simulink model "poleplacement_2"  (Simulink 7.8)
settings: Solver=ode1  StartTime=0.0  StopTime=inf  FixedStep=0.002  RelTol=1e-3
values from neighbouring files (symbols this model uses):
  k_1 = K(1)    [lqr_lab.m]
  k_2 = K(2)    [lqr_lab.m]
  k_3 = K(3)    [lqr_lab.m]
  k_4 = K(4)    [lqr_lab.m]
  Kth = 0.00153    [params.m]
  Kx = 2.28E-5    (= 2.28e-05)    [params.m]
undefined symbols (not defined in the file or in its folder): HIL
libraries: quarc_library x3, dsparch4 x2, simulink_extras x1
settings Model: Creator=dlavoi14  LastModifiedBy=dlavoi14  SimulationMode=external  ExtModeTrigDuration=5000
settings SolverCC: PositivePriorityOrder=on
settings RTWCC: SystemTargetFile=quarc_win64.tlc  TemplateMakefile=quarc_default_tmf  Description=QUARC Win64 Target  ProcessScript=quarc_win64_make_rtw_hook
settings STFCustomTargetCC: TargetPreCompLibLocation=C:\PROGRA~3\QUARC\lib\2011b\win64\release  SystemTargetFile=quarc_win64.tlc
settings GRTTargetCC: TargetPreCompLibLocation=C:\PROGRA~3\QUARC\lib\2011b\win64\release  ParMdlRefBuildCompliant=off  CompOptLevelCompliant=off  ConcurrentExecutionCompliant=off  MatFileLogging=off  ExtMode=on  ExtModeMexFile=quarc_comm

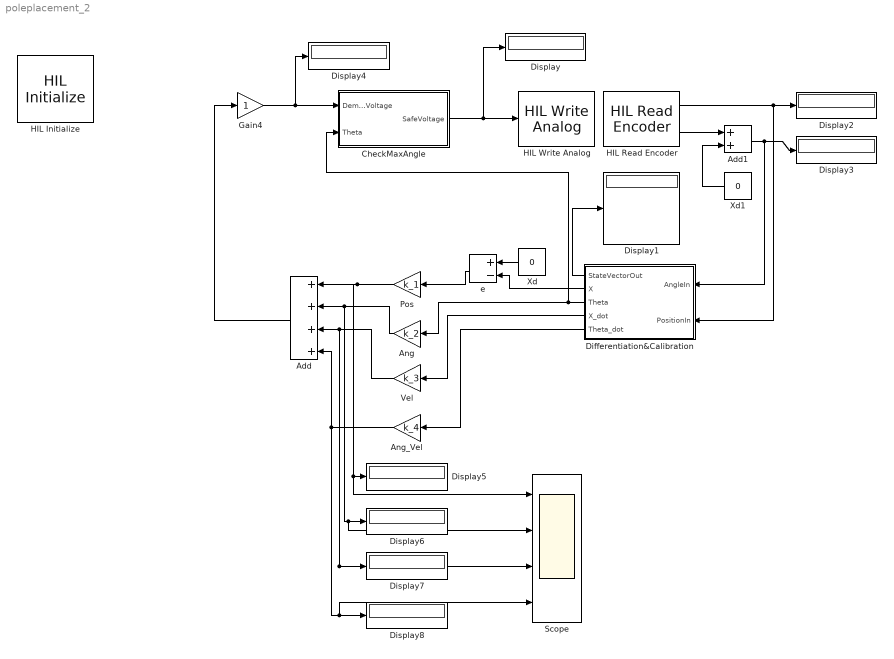
== system poleplacement_2 ==
  Add : Sum  Inputs=++++
  Add1 : Sum
  Ang : Gain  Gain=k_2
  Ang_Vel : Gain  Gain=k_4
  CheckMaxAngle : Subsystem
  Differentiation&Calibration : Subsystem
  Display{,1..8} (9 alike) : Display
  Gain4 : Gain
  HIL Initialize : quarc_library/Data Acquisition/Generic/Configuration/HIL Initialize  Priority=-99  object_name=HIL-1  board_type=q4  board_number=0  exclusive=off  active=off  hardware_clocks=[0:1]  clock_modes=[0 0]  initial_clock_frequencies=[]  set_clock_params_at_start=on  set_clock_params_at_switch_in=off  set_clock_frequencies_at_start=off  set_clock_frequencies_at_switch_in=off  analog_input_channels=[0:3]  analog_input_maximums=10  analog_input_minimums=-10  set_analog_input_params_at_start=off  set_analog_input_params_at_switch_in=off  analog_output_channels=[0:3]  analog_output_maximums=[10]  analog_output_minimums=[-10]  initial_analog_outputs=[0]  final_analog_outputs=[0]  watchdog_analog_outputs=0  set_analog_output_params_at_start=on  set_analog_output_params_at_switch_in=off  set_analog_outputs_at_start=on  set_analog_outputs_at_switch_in=off  set_analog_outputs_at_terminate=on  set_analog_outputs_at_switch_out=off  set_analog_outputs_on_watchdog=off  digital_input_channels=[]  digital_output_channels=[]  digital_output_configuration=[]  initial_digital_outputs=[1]  final_digital_outputs=[1]  watchdog_digital_outputs=[2]  set_digital_output_params_at_start=off  set_digital_output_params_at_switch_in=off  set_digital_outputs_at_start=on  set_digital_outputs_at_switch_in=off  set_digital_outputs_at_terminate=on  set_digital_outputs_at_switch_out=off  set_digital_outputs_on_watchdog=off  encoder_channels=[0:3]  quadrature=[4]  encoder_filter_frequency=(1/60e-9)/1  initial_encoder_counts=[0]  set_encoder_params_at_start=on  set_encoder_params_at_switch_in=off  set_encoder_counts_at_start=on  set_encoder_counts_at_switch_in=off  pwm_channels=[]  pwm_modes=[0]  pwm_frequency=(1/60e-9)/1024  pwm_configuration=[]  pwm_alignment=[]  pwm_polarity=[]  pwm_leading_deadband=[]  pwm_trailing_deadband=[]  initial_pwm_outputs=[0]  final_pwm_outputs=[0]  watchdog_pwm_outputs=[]  set_pwm_params_at_start=on  set_pwm_params_at_switch_in=off  set_pwm_outputs_at_start=on  set_pwm_outputs_at_switch_in=off  set_pwm_outputs_at_terminate=on  set_pwm_outputs_at_switch_out=off  set_pwm_outputs_on_watchdog=off  other_output_channels=[]  initial_other_outputs=[]  final_other_outputs=[]  watchdog_other_outputs=[]  set_other_outputs_at_start=off  set_other_outputs_at_switch_in=off  set_other_outputs_at_terminate=off  set_other_outputs_at_switch_out=off  set_other_outputs_on_watchdog=off
  HIL Read Encoder : quarc_library/Data Acquisition/Generic/Immediate I//O/HIL Read Encoder  object_name=HIL-1  channels=[0:1]  sample_time=qc_get_step_size  active=on  vector_output=off  data_type_mode=Inherit via back propagation  data_type=double
  HIL Write Analog : quarc_library/Data Acquisition/Generic/Immediate I//O/HIL Write Analog  object_name=HIL-1  channels=0  sample_time=-1  active=off  vector_input=off
  Pos : Gain  Gain=k_1
  Scope : Scope  NumInputPorts=4
      settings: YMin=-5~-80~-22.5~-80  YMax=6~90~22.5~60
  Vel : Gain  Gain=k_3
  Xd : Constant  Value=0
  Xd1 : Constant  Value=0
  e : Sum  Inputs=+-
  wires:
  CheckMaxAngle/1(SafeVoltage) -> Display/1, HIL Write Analog/1
  HIL Read Encoder/1 -> Differentiation&Calibration/2(PositionIn), Display2/1
  Differentiation&Calibration/3(Theta) -> Ang/1, CheckMaxAngle/2(Theta)
  Differentiation&Calibration/4(X_dot) -> Vel/1
  Differentiation&Calibration/5(Theta_dot) -> Ang_Vel/1
  Pos/1 -> Add/1, Display5/1, Scope/1
  Ang/1 -> Add/2, Display6/1, Scope/2
  Vel/1 -> Add/3, Display7/1, Scope/3
  Ang_Vel/1 -> Add/4, Display8/1, Scope/4
  Add/1 -> Gain4/1
  Gain4/1 -> Display4/1, CheckMaxAngle/1(DemandedControlVoltage)
  Differentiation&Calibration/2(X) -> e/2
  e/1 -> Pos/1
  Xd/1 -> e/1
  HIL Read Encoder/2 -> Add1/1
  Xd1/1 -> Add1/2
  Add1/1 -> Display3/1, Differentiation&Calibration/1(AngleIn)
  Differentiation&Calibration/1(StateVectorOut) -> Display1/1

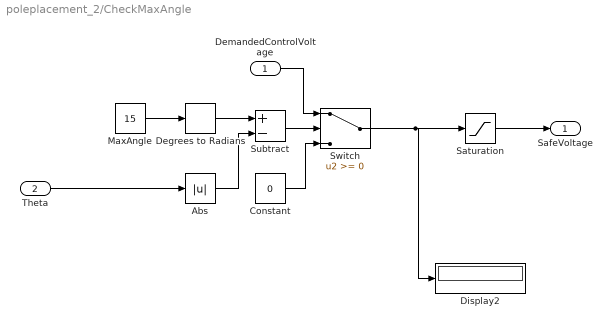
== system poleplacement_2/CheckMaxAngle ==
  DemandedControlVoltage : Inport
  Theta : Inport  Port=2
  Abs : Abs
  Constant : Constant  Value=0
  Degrees to Radians : simulink_extras/Transformations/Degrees to Radians
  Display2 : Display
  MaxAngle : Constant  Value=15
  Saturation : Saturate  UpperLimit=5  LowerLimit=-5
  Subtract : Sum  Inputs=+-
  Switch : Switch
  SafeVoltage : Outport
  wires:
  DemandedControlVoltage/1 -> Switch/1
  Constant/1 -> Switch/3
  Switch/1 -> Display2/1, Saturation/1
  MaxAngle/1 -> Degrees to Radians/1
  Theta/1 -> Abs/1
  Degrees to Radians/1 -> Subtract/1
  Subtract/1 -> Switch/2
  Abs/1 -> Subtract/2
  Saturation/1 -> SafeVoltage/1

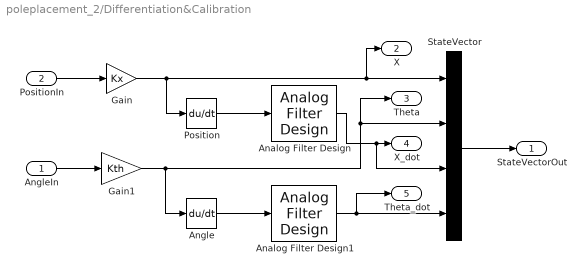
== system poleplacement_2/Differentiation&Calibration ==
  AngleIn : Inport
  PositionIn : Inport  Port=2
  Analog Filter Design : dsparch4/Analog Filter Design  method=Butterworth  filttype=Lowpass  N=8  Wlo=30  Whi=80  Rp=2  Rs=40
  Analog Filter Design1 : dsparch4/Analog Filter Design  method=Butterworth  filttype=Lowpass  N=8  Wlo=30  Whi=80  Rp=2  Rs=40
  Angle : Derivative
  Gain : Gain  Gain=Kx
  Gain1 : Gain  Gain=Kth
  Position : Derivative
  StateVector : Concatenate  NumInputs=4  Mode=Vector
  StateVectorOut : Outport
  X : Outport  Port=2
  Theta : Outport  Port=3
  X_dot : Outport  Port=4
  Theta_dot : Outport  Port=5
  wires:
  StateVector/1 -> StateVectorOut/1
  AngleIn/1 -> Gain1/1
  PositionIn/1 -> Gain/1
  Gain/1 -> Position/1, StateVector/1, X/1
  Gain1/1 -> Angle/1, StateVector/2, Theta/1
  Angle/1 -> Analog Filter Design1/1
  Analog Filter Design1/1 -> StateVector/4, Theta_dot/1
  Position/1 -> Analog Filter Design/1
  Analog Filter Design/1 -> StateVector/3, X_dot/1
